simulink model "ModulateurSigmaDelta"  (R2015a)
settings: Solver=ode3  StartTime=0.0  StopTime=Tsim  FixedStep=TsR  RelTol=1e-3
values from neighbouring files (symbols this model uses):
  nu0 = 10    [mConvertisseurSigmaDelta.m]    (also in mModulateurSigmaDelta.m)
settings Model: ExtModeTrigMode=oneshot  ExtModeArmWhenConnect=off  Creator=gscorlet  LastModifiedBy=julo
settings DataIOCC: LimitDataPoints=off  SignalLoggingSaveFormat=ModelDataLogs
settings OptimizationCC: BlockReduction=off  BooleanDataType=off  ExpressionDepthLimit=2147483647
settings DebuggingCC: SaveWithParameterizedLinksMsg=none  UnderspecifiedInitializationDetection=Classic  MergeDetectMultiDrivingBlocksExec=none  SignalResolutionControl=TryResolveAllWithWarning  MultiTaskDSMMsg=warning  MultiTaskCondExecSysMsg=none  FcnCallInpInsideContextMsg=UseLocalSettings  StateNameClashWarn=warning
settings HardwareCC: TargetUnknown=on
settings GRTTargetCC: CombineOutputUpdateFcns=off  GRTInterface=on

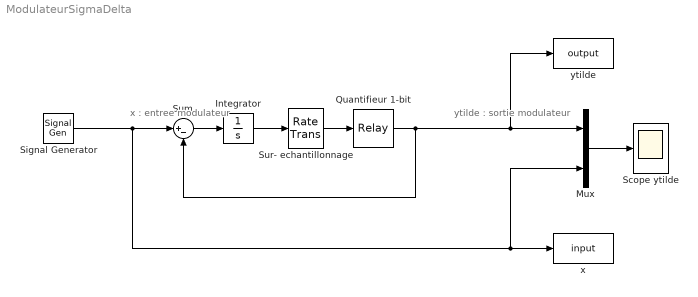
== system ModulateurSigmaDelta ==
  note: x : entree
      | modulateur
  note: ytilde : sortie
      | modulateur
  Integrator : Integrator
  Mux : Mux  Inputs=2
  Quantifieur 1-bit : Relay  OffSwitchValue=-eps  OffOutputValue=-1
  Scope ytilde : Scope
      settings: TimeRange=1  YMin=-1.5  YMax=1.5  SampleInput=on
  Signal Generator : SignalGenerator  Frequency=nu0
  Sum : Sum  Inputs=|+-  SaturateOnIntegerOverflow=on  InputSameDT=on  OutDataTypeStr=Inherit: Same as first input
  Sur- echantillonnage : RateTransition  OutPortSampleTime=TsR
  x : ToWorkspace  VariableName=input  SaveFormat=Timeseries  SampleTime=-1
  ytilde : ToWorkspace  VariableName=output  SaveFormat=Timeseries  SampleTime=-1
  wires:
  Integrator/1 -> Sur- echantillonnage/1
  Sum/1 -> Integrator/1
  Signal Generator/1 -> Sum/1, x/1, Mux/2
  Mux/1 -> Scope ytilde/1
  Sur- echantillonnage/1 -> Quantifieur 1-bit/1
  Quantifieur 1-bit/1 -> Sum/2, Mux/1, ytilde/1
